simulink model "three_tank_model"  (R2022b)
settings: Solver=VariableStepAuto  StartTime=0.0  StopTime=10.0  RelTol=1e-3
settings Model: Creator=varun  LastModifiedBy=varun

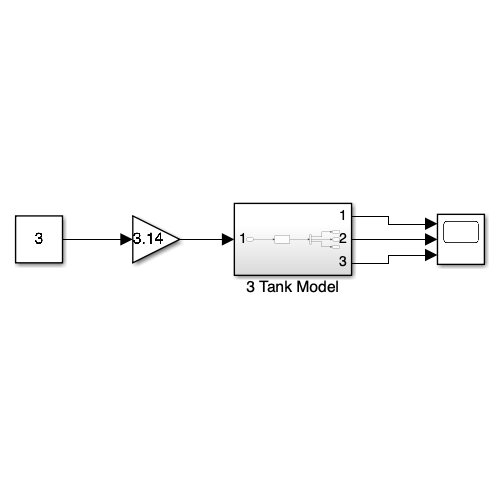
[thumbnail: Simulink's stored preview of the top-level diagram]
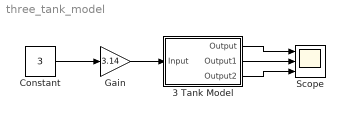
== system three_tank_model ==
  3 Tank Model : Subsystem
  Constant : Constant  Value=3
  Gain : Gain  Gain=3.14
  Scope : Scope  NumInputPorts=3
  wires:
  Constant/1 -> Gain/1
  Gain/1 -> 3 Tank Model/1(Input)
  3 Tank Model/1(Output) -> Scope/1
  3 Tank Model/2(Output1) -> Scope/2
  3 Tank Model/3(Output2) -> Scope/3

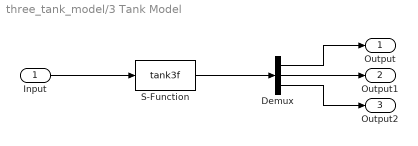
== system three_tank_model/3 Tank Model ==
  Input : Inport
  Demux : Demux  Outputs=3
  S-Function : S-Function  FunctionName=tank3f  SFunctionDeploymentMode=off  EnableBusSupport=off
  Output : Outport
  Output1 : Outport  Port=2
  Output2 : Outport  Port=3
  wires:
  S-Function/1 -> Demux/1
  Input/1 -> S-Function/1
  Demux/1 -> Output/1
  Demux/3 -> Output2/1
  Demux/2 -> Output1/1
